simulink model "Ex1"  (R2023a)
settings: Solver=VariableStepAuto  StartTime=0.0  StopTime=600  RelTol=1e-3
libraries: slpidlib x1
settings Model: Creator=gutoc  LastModifiedBy=gutoc

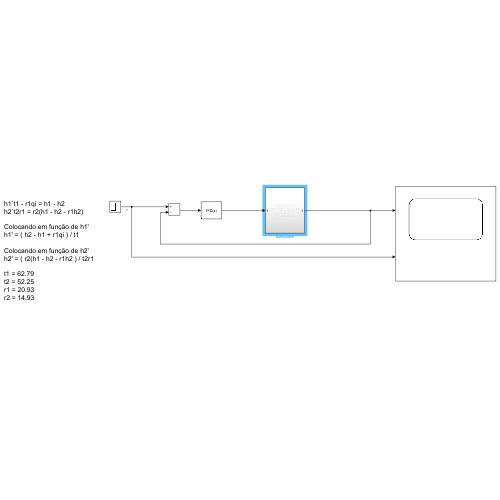
[thumbnail: Simulink's stored preview of the top-level diagram]
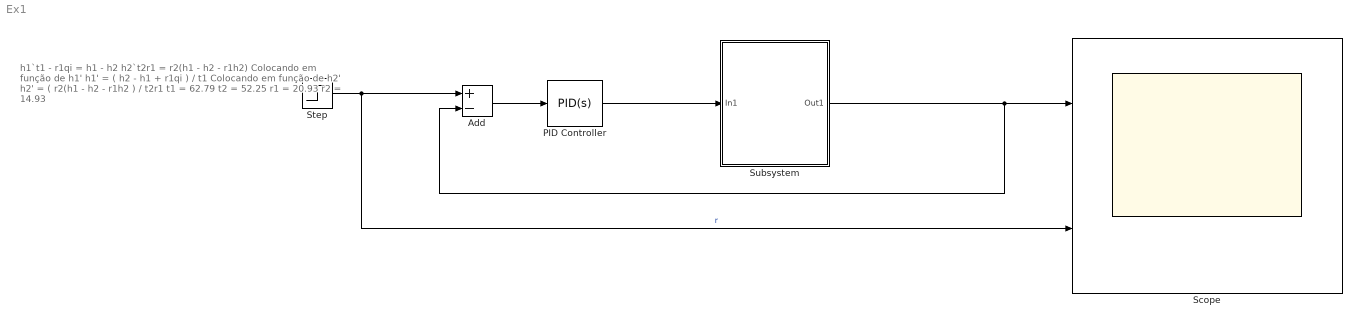
== system Ex1 ==
  note: h1`t1 - r1qi = h1 - h2
      | h2`t2r1 = r2(h1 - h2 - r1h2)
      |
      | Colocando em função de h1'
      | h1' = ( h2 - h1 + r1qi ) / t1
      |
      | Colocando em função de h2'
      | h2' = ( r2(h1 - h2 - r1h2 ) / t2r1
      |
      | t1 = 62.79
      | t2 = 52.25
      | r1 = 20.93
      | r2 = 14.93
  Add : Sum  Inputs=+-
  PID Controller : slpidlib/PID Controller  Controller=PID  Form=Parallel  TimeDomain=Continuous-time  UseExternalTs=off  SampleTime=-1  IntegratorMethod=Forward Euler  FilterMethod=Forward Euler  ControllerParametersSource=internal  P=0.3  I=0.003  UseKiTs=off  D=5.75  N=100  UseFilter=on  TunerSelectOption=Transfer Function Based (PID Tuner App)  InitialConditionSource=internal  InitialConditionForIntegrator=0  InitialConditionForFilter=0  DifferentiatorICPrevScaledInput=0  ExternalReset=none  TrackingMode=off  Kt=1  LimitOutput=off  SatLimitsSource=internal  UpperSaturationLimit=inf  LowerSaturationLimit=-inf  LinearizeAsGain=on  AntiWindupMode=none  Kb=1  LimitIntegrator=off  UpperIntegratorSaturationLimit=inf  LowerIntegratorSaturationLimit=-inf  POutMin=[]  POutMax=[]  IOutMin=[]  IOutMax=[]  DOutMin=[]  DOutMax=[]  NOutMin=[]  NOutMax=[]  SumOutMin=[]  SumOutMax=[]  SaturationOutMin=[]  SaturationOutMax=[]  PParamMin=[]  PParamMax=[]  IParamMin=[]  IParamMax=[]  DParamMin=[]  DParamMax=[]  NParamMin=[]  NParamMax=[]  KbParamMin=[]  KbParamMax=[]  KtParamMin=[]  KtParamMax=[]  KbOutMin=[]  KbOutMax=[]  KtOutMin=[]  KtOutMax=[]  IntegratorOutMin=[]  IntegratorOutMax=[]  FilterOutMin=[]  FilterOutMax=[]  SumI1OutMin=[]  SumI1OutMax=[]  SumI2OutMin=[]  SumI2OutMax=[]  SumI3OutMin=[]  SumI3OutMax=[]  SumI4OutMin=[]  SumI4OutMax=[]  SumDOutMin=[]  SumDOutMax=[]  DifferentiatorOutMin=[]  DifferentiatorOutMax=[]  FilterDiffOutCoefMin=[]  FilterDiffOutCoefMax=[]  ReciprocalOutMin=[]  ReciprocalOutMax=[]  SumDenOutMin=[]  SumDenOutMax=[]  SumNumOutMin=[]  SumNumOutMax=[]  DivideOutMin=[]  DivideOutMax=[]  UdiffTsProdOutMin=[]  UdiffTsProdOutMax=[]  NTsProdOutMin=[]  NTsProdOutMax=[]  UintegralTsProdOutMin=[]  UintegralTsProdOutMax=[]  UngainTsProdOutMin=[]  UngainTsProdOutMax=[]  ClampingZeroOutDataTypeStr=Inherit: Inherit via back propagation  ClampingZeroOutMin=[]  ClampingZeroOutMax=[]  FilterDenConstantOutDataTypeStr=Inherit: Inherit via back propagation  FilterDenConstantOutMin=[]  FilterDenConstantOutMax=[]  PCopyOutDataTypeStr=Inherit: Inherit via back propagation  PCopyOutMin=[]  PCopyOutMax=[]  NCopyOutDataTypeStr=Inherit: Inherit via back propagation  NCopyOutMin=[]  NCopyOutMax=[]  IntegratorContinuousStateAttributes=''  IntegratorStateMustResolveToSignalObject=off  IntegratorRTWStateStorageClass=Auto  FilterContinuousStateAttributes=''  FilterStateMustResolveToSignalObject=off  FilterRTWStateStorageClass=Auto  ParallelPVariant=InternalParameters  IdealPVariant=Disabled  IVariant=InternalParameters  DVariant=InternalParameters  IntegratorVariant=Continuous  SatVariant=Disabled  AWVariant=Passthrough  PCopyVariant=Disabled  TRVariant=Disabled  FdbkBlocksVariant=Forward  IdealPFdbkVariant=Disabled  SatFdbkVariant=Disabled  DerivativeFilterVariant=ContFilter  NVariant=InternalParameters  NCopyVariant=Disabled  FilterICVariant=InternalICsFilter  IntegratorICVariant=InternalICs  ExternalResetVariant=Disabled  TRSumVariant=Passthrough  SumFdbkVariant=Disabled  SumVariant=Sum_PID  TsampFilterVariant=InternalTs  TsampNgainVariant=Passthrough  TsampIntegralVariant=Disabled_SignalSpec  ExternalSaturationOutDataTypeStr=Inherit: Same as second input
  Scope : Scope  NumInputPorts=2
  Step : Step  SampleTime=0
  Subsystem : Subsystem
  wires:
  Step/1 -> Add/1, Scope/2  "r"
  Add/1 -> PID Controller/1
  PID Controller/1 -> Subsystem/1(In1)
  Subsystem/1(Out1) -> Scope/1, Add/2

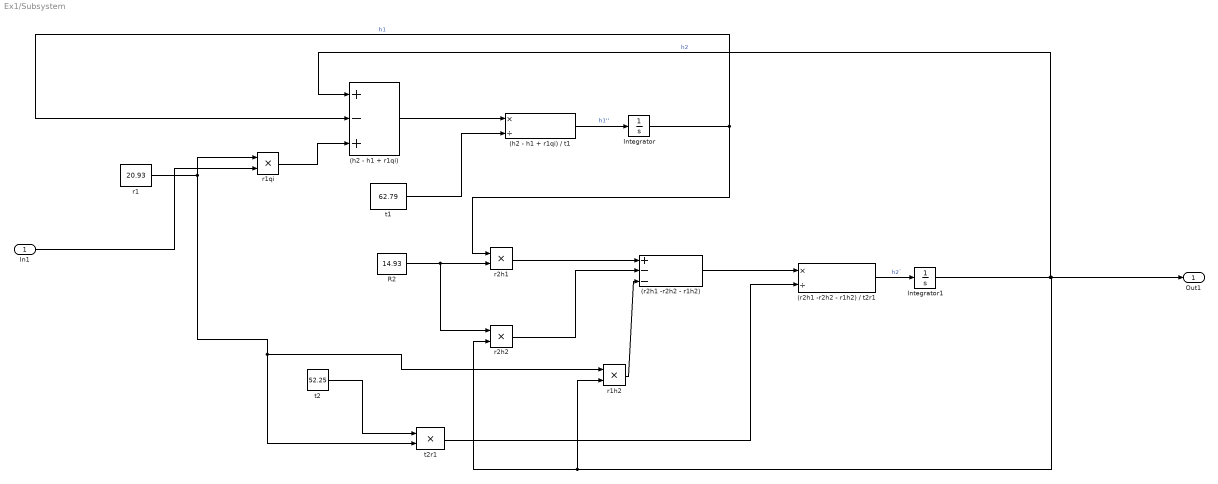
== system Ex1/Subsystem ==
  In1 : Inport
  (h2 - h1 + r1qi) : Sum  Inputs=+-+
  (h2 - h1 + r1qi) / t1 : Product  Inputs=*/
  (r2h1 -r2h2 - r1h2) : Sum  Inputs=+--
  (r2h1 -r2h2 - r1h2) / t2r1 : Product  Inputs=*/
  Integrator : Integrator
  Integrator1 : Integrator
  R2 : Constant  Value=14.93
  r1 : Constant  Value=20.93
  r1h2 : Product
  r1qi : Product
  r2h1 : Product
  r2h2 : Product
  t1 : Constant  Value=62.79
  t2 : Constant  Value=52.25
  t2r1 : Product
  Out1 : Outport
  wires:
  r1h2/1 -> (r2h1 -r2h2 - r1h2)/3
  r2h2/1 -> (r2h1 -r2h2 - r1h2)/2
  (h2 - h1 + r1qi)/1 -> (h2 - h1 + r1qi) / t1/1
  r2h1/1 -> (r2h1 -r2h2 - r1h2)/1
  r1/1 -> r1h2/1, t2r1/2, r1qi/1
  t1/1 -> (h2 - h1 + r1qi) / t1/2
  R2/1 -> r2h2/1, r2h1/2
  (r2h1 -r2h2 - r1h2) / t2r1/1 -> Integrator1/1  "h2`"
  Integrator1/1 -> (h2 - h1 + r1qi)/1, Out1/1, r1h2/2, r2h2/2  "h2"
  t2/1 -> t2r1/1
  (r2h1 -r2h2 - r1h2)/1 -> (r2h1 -r2h2 - r1h2) / t2r1/1
  r1qi/1 -> (h2 - h1 + r1qi)/3
  (h2 - h1 + r1qi) / t1/1 -> Integrator/1  "h1''"
  t2r1/1 -> (r2h1 -r2h2 - r1h2) / t2r1/2
  In1/1 -> r1qi/2
  Integrator/1 -> (h2 - h1 + r1qi)/2, r2h1/1  "h1"
